simulink model "stepper_motor"  (R2014a)
settings: Solver=VariableStepDiscrete  StartTime=0.0  StopTime=1  RelTol=1e-3
undefined symbols (not defined in the file or in its folder): DiscIntNeverNeededParam, flc_pid3
libraries: powerlib x7, fuzblock x1
settings Model: Creator=krish  LastModifiedBy=krish

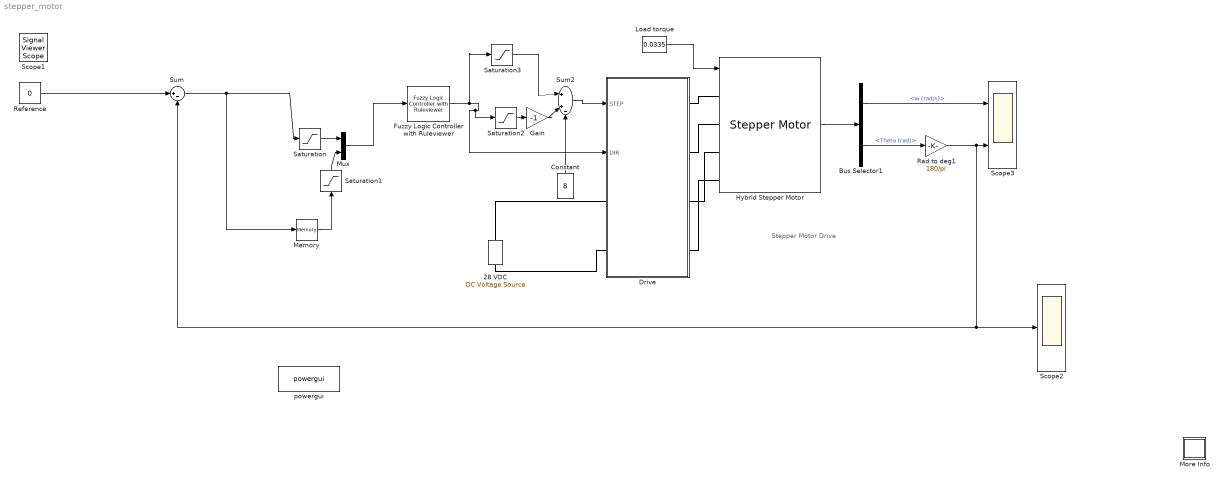
== system stepper_motor ==
  note: Stepper Motor Drive
  28 VDC : powerlib/Electrical Sources/DC Voltage Source  Amplitude=28  Measurements=None
  Bus Selector1 : BusSelector  OutputSignals=w (rad/s),Theta (rad)
  Constant : Constant  Value=8
  Drive : Subsystem  mask{Iref=2, step=500, Ts=1e-6}
      mask prompts: Iref "Phase current (A)"; step "Stepping rate (step/s)"; Ts "Sampling time (s)"
      mask init:
      | Nstep=round(1/step/Ts);
  Fuzzy Logic Controller with Ruleviewer : fuzblock/Fuzzy Logic  Controller  with Ruleviewer  fismatrix=[flc_pid3]  Ts=2
  Gain : Gain  Gain=-1
  Hybrid Stepper Motor : powerlib/Machines/Stepper Motor  MotorType=Permanent-magnet / Hybrid  NumberOfPhases_1=2  NumberOfPhases_2=3  PresetModel_1=<empty>  PresetModel_2=<empty>  L=1.4e-3  Lmax=10e-3  Lmin=2e-3  R=0.7  Step_angle=1.8  Psim=0.005  Tdm=0.002  J=1.2e-7  B=1e-7  w0=0  pos0=-10  TsPowergui=0  TsBlock=-1
  Load torque : Constant  Value=0.0335
  Memory : Memory
  More Info : Subsystem
      settings: OpenFcn=showdemo(bdroot(gcb))
      mask Display: disp('?')
  Mux : Mux  Inputs=2
  Rad to deg1 : Gain  Gain=180/pi
  Reference : Constant  Value=0
  Saturation : Saturate  UpperLimit=50  LowerLimit=-50
  Saturation1 : Saturate  UpperLimit=5  LowerLimit=-5
  Saturation2 : Saturate  UpperLimit=5  LowerLimit=-5
  Saturation3 : Saturate  UpperLimit=10  LowerLimit=-10
  Scope2 : Scope
      settings: TimeRange=0.2  YMin=-10.25  YMax=-7  SaveName=VIX
  Scope3 : Scope  NumInputPorts=2
      settings: TimeRange=0.2  YMin=-4~-7.28  YMax=4~-7.2715  SaveName=VIX1
  Sum : Sum  Inputs=|+-
  Sum2 : Sum  Inputs=|++-
  powergui : powerlib/powergui  SimulationMode=Discrete  SolverType=Tustin  SampleTime=1e-6  frequency=60  SPID=off  DisableSnubberDevices=off  DisableRonSwitches=off  DisableVfSwitches=off  SwTol=0  Interpol=off  DisplayEquations=off  Ts=0  methode=off  frequencyindice=0  Pbase=100e6  ErrMax=1e-4  Iterations=50  UnitsV=kV  UnitsW=MW  FunctionMessages=off  echomessages=off  HookPort=off  EnableUseOfTLC=off  x0status=blocks  RestoreLinks=warning  ResistiveCurrentMeasurement=off  Frange=[0:2:500]  Ylog=off  Xlog=on  ShowGrid=off  save=off  variable=ZData  structure=0  ZoomFFT=on  StartTime=0.0  cycles=1  DisplayStyle=1  fundamental=60  FreqAxis=off  MaxFrequency=1000  frequencyindicesteady=1  RmsSteady=1  display=off
  Scope1 : SignalViewerScope  IOType=viewer  RefreshTime=0.035000
  wires:
  Load torque/1 -> Hybrid Stepper Motor/1
  Fuzzy Logic Controller with Ruleviewer/1 -> Saturation2/1, Drive/2(DIR), Saturation3/1
  Mux/1 -> Fuzzy Logic Controller with Ruleviewer/1
  Sum/1 -> Memory/1, Saturation/1
  Memory/1 -> Saturation1/1
  Bus Selector1/1 -> Scope3/1  "<w (rad/s)>"
  Bus Selector1/2 -> Rad to deg1/1  "<Theta (rad)>"
  Hybrid Stepper Motor/1 -> Bus Selector1/1
  Rad to deg1/1 -> Scope2/1, Sum/2, Scope3/2
  Reference/1 -> Sum/1
  Saturation/1 -> Mux/1
  Saturation1/1 -> Mux/2
  Saturation2/1 -> Gain/1
  Gain/1 -> Sum2/2
  Saturation3/1 -> Sum2/1
  Constant/1 -> Sum2/3
  Sum2/1 -> Drive/1(STEP)
  connections:
  Drive/RConn2 -- Hybrid Stepper Motor/LConn2
  Drive/RConn3 -- Hybrid Stepper Motor/LConn3
  Drive/RConn1 -- Hybrid Stepper Motor/LConn1
  Drive/LConn2 -- 28 VDC/LConn1
  28 VDC/RConn1 -- Drive/LConn1
  Drive/RConn4 -- Hybrid Stepper Motor/LConn4

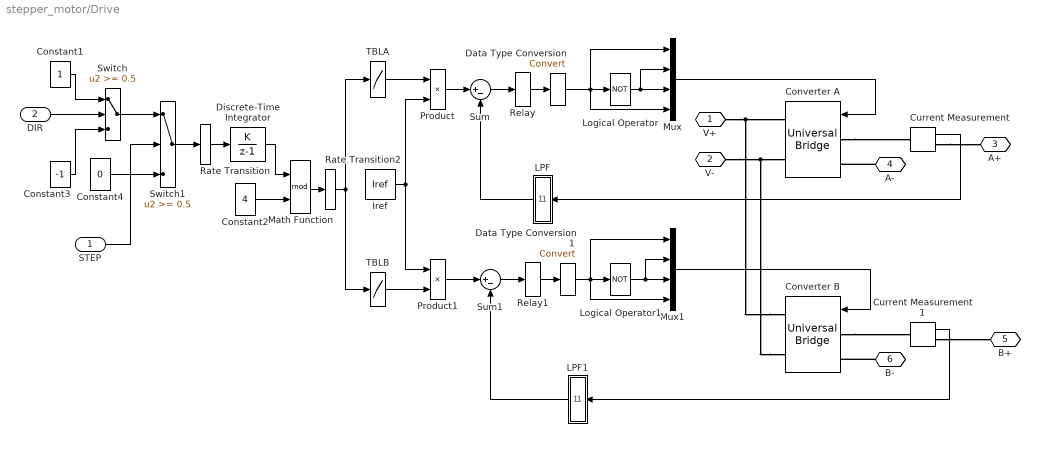
== system stepper_motor/Drive ==
  STEP : Inport
  DIR : Inport  Port=2
  Constant1 : Constant  SampleTime=Ts
  Constant2 : Constant  Value=4  SampleTime=Nstep*Ts
  Constant3 : Constant  Value=-1  SampleTime=Ts
  Constant4 : Constant  Value=0  SampleTime=Ts
  Converter A : powerlib/Power Electronics/Universal Bridge  Arms=2  SnubberResistance=10000  SnubberCapacitance=inf  Device=MOSFET / Diodes  Ron=1e-3*10  Lon=0  ForwardVoltages="[  0  0  ]"  ForwardVoltage=0  GTOparameters=[ 10e-6 , 20e-6 ]  IGBTparameters=[ 0.5e-6 , 0.5e-6 ]  Measurements=None  Measurements_2=None  converterType=Rectifier
  Converter B : powerlib/Power Electronics/Universal Bridge  Arms=2  SnubberResistance=10000  SnubberCapacitance=inf  Device=MOSFET / Diodes  Ron=1e-3*10  Lon=0  ForwardVoltages="[  0  0  ]"  ForwardVoltage=0  GTOparameters=[ 10e-6 , 20e-6 ]  IGBTparameters=[ 0.5e-6 , 0.5e-6 ]  Measurements=None  Measurements_2=None  converterType=Rectifier
  Current Measurement : powerlib/Measurements/Current Measurement  PhasorSimulation=off  OutputType=Complex  PSBequivalent=0
  Current Measurement1 : powerlib/Measurements/Current Measurement  PhasorSimulation=off  OutputType=Complex  PSBequivalent=0
  Data Type Conversion : DataTypeConversion
  Data Type Conversion1 : DataTypeConversion
  Discrete-Time Integrator : DiscreteIntegrator  IntegratorMethod=Accumulation: Forward Euler  SampleTime=Nstep*Ts  ICPrevOutput=DiscIntNeverNeededParam  ICPrevScaledInput=DiscIntNeverNeededParam
  Iref : Constant  Value=Iref  SampleTime=Ts
  LPF : Subsystem  mask{fc=10000, Ts=Ts}
      mask prompts: fc "Cut-off frequency (Hz)"; Ts "Sampling time (s)"
      mask init:
      | % fa=tf(1,[1/2/pi/fc 1]);
      | % fn=c2d(fa,Ts);
      | % [NN,DD]=tfdata(fn,'v')
      | 
      | NN = [ 0,0.0609];
      | DD = [1.0000,-0.9391];
  LPF1 : Subsystem  mask{fc=10000, Ts=Ts}
      mask prompts: fc "Cut-off frequency (Hz)"; Ts "Sampling time (s)"
      mask init:
      | % fa=tf(1,[1/2/pi/fc 1]);
      | % fn=c2d(fa,Ts);
      | % [NN,DD]=tfdata(fn,'v')
      | 
      | NN = [ 0,0.0609];
      | DD = [1.0000,-0.9391];
  Logical Operator : Logic  Operator=NOT  AllPortsSameDT=off  OutDataTypeStr=boolean
  Logical Operator1 : Logic  Operator=NOT  AllPortsSameDT=off  OutDataTypeStr=boolean
  Math Function : Math  Operator=mod  SampleTime=Nstep*Ts  SaturateOnIntegerOverflow=on
  Mux : Mux
  Mux1 : Mux
  Product : Product  RndMeth=Zero
  Product1 : Product  RndMeth=Zero
  Rate Transition : RateTransition
  Rate Transition2 : RateTransition
  Relay : Relay  OnSwitchValue=0.01  OffSwitchValue=-0.01
  Relay1 : Relay  OnSwitchValue=0.01  OffSwitchValue=-0.01  OutDataTypeStr=Inherit: Inherit via back propagation
  Sum : Sum  Inputs=|+-  OutDataTypeStr=Inherit: Same as first input
  Sum1 : Sum  Inputs=|+-  OutDataTypeStr=Inherit: Same as first input
  Switch : Switch  Threshold=0.5  ZeroCross=off  SampleTime=Ts
  Switch1 : Switch  Threshold=0.5  ZeroCross=off  SampleTime=Ts
  TBLA : Lookup  InputValues=[0:3]  Table=[1 0 -1 0]  SampleTime=Ts
  TBLB : Lookup  InputValues=[0:3]  Table=[0 1 0 -1]  SampleTime=Ts
  V+ : PMIOPort  Port=1  Side=Left
  V- : PMIOPort  Port=2  Side=Left
  A+ : PMIOPort  Port=3  Side=Right
  A- : PMIOPort  Port=4  Side=Right
  B+ : PMIOPort  Port=5  Side=Right
  B- : PMIOPort  Port=6  Side=Right
  wires:
  Constant4/1 -> Switch1/3
  Switch1/1 -> Rate Transition/1
  Switch/1 -> Switch1/1
  STEP/1 -> Switch1/2
  DIR/1 -> Switch/2
  Rate Transition2/1 -> TBLB/1, TBLA/1
  Math Function/1 -> Rate Transition2/1
  Product1/1 -> Sum1/1
  Product/1 -> Sum/1
  Rate Transition/1 -> Discrete-Time Integrator/1
  Constant3/1 -> Switch/3
  Constant1/1 -> Switch/1
  Discrete-Time Integrator/1 -> Math Function/1
  Constant2/1 -> Math Function/2
  Iref/1 -> Product1/1, Product/2
  TBLB/1 -> Product1/2
  TBLA/1 -> Product/1
  LPF1/1(O) -> Sum1/2
  LPF/1(O) -> Sum/2
  Data Type Conversion1/1 -> Mux1/4, Mux1/1, Logical Operator1/1
  Data Type Conversion/1 -> Logical Operator/1, Mux/4, Mux/1
  Current Measurement1/1 -> LPF1/1(I)
  Sum1/1 -> Relay1/1
  Mux1/1 -> Converter B/1
  Logical Operator1/1 -> Mux1/2, Mux1/3
  Relay1/1 -> Data Type Conversion1/1
  Mux/1 -> Converter A/1
  Logical Operator/1 -> Mux/2, Mux/3
  Relay/1 -> Data Type Conversion/1
  Current Measurement/1 -> LPF/1(I)
  Sum/1 -> Relay/1
  connections:
  Converter B/RConn2 -- Converter A/RConn2 -- V-/RConn1
  Converter B/RConn1 -- Converter A/RConn1 -- V+/RConn1
  Current Measurement1/RConn1 -- B+/RConn1
  Converter B/LConn1 -- Current Measurement1/LConn1
  Current Measurement/RConn1 -- A+/RConn1
  Converter A/LConn1 -- Current Measurement/LConn1
  B-/RConn1 -- Converter B/LConn2
  A-/RConn1 -- Converter A/LConn2

== system stepper_motor/More Info ==

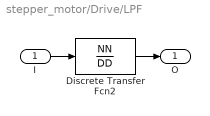
== system stepper_motor/Drive/LPF ==
  I : Inport
  Discrete Transfer Fcn2 : DiscreteTransferFcn  Numerator=NN  Denominator=DD  SampleTime=Ts
  O : Outport
  wires:
  Discrete Transfer Fcn2/1 -> O/1
  I/1 -> Discrete Transfer Fcn2/1

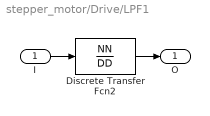
== system stepper_motor/Drive/LPF1 ==
  I : Inport
  Discrete Transfer Fcn2 : DiscreteTransferFcn  Numerator=NN  Denominator=DD  SampleTime=Ts
  O : Outport
  wires:
  I/1 -> Discrete Transfer Fcn2/1
  Discrete Transfer Fcn2/1 -> O/1
